simulink model "Standalone_AutoTuner"  (R2025b)
settings: Solver=FixedStepDiscrete  StartTime=0.0  StopTime=20  FixedStep=1e-4  MaxStep=1e-4  RelTol=1e-3  EnableMultiTasking=on
settings Model: SimulationMode=software-in-the-loop (sil)  CodeVerificationMode=processor-in-the-loop (pil)  Creator=Harish  LastModifiedBy=Harish
settings OptimizationCC: DefaultParameterBehavior=Inlined  EnhancedBackFolding=on  PassReuseOutputArgsAs=Individual arguments  ZeroExternalMemoryAtStartup=off  ZeroInternalMemoryAtStartup=off  MaxStackSize=64  OptimizeBlockOrder=speed  DifferentSizesBufferReuse=on  OptimizationCustomize=off  EfficientTunableParamExpr=on
settings DebuggingCC: ParameterTunabilityLossMsg=error
settings HardwareCC: ProdBitPerPointer=32.0  ProdBitPerSizeT=32.0  ProdBitPerPtrDiffT=32.0  ProdLargestAtomicInteger=Long  ProdLargestAtomicFloat=Double  ProdWordSize=32.0  ProdLongLongMode=on  ProdHWDeviceType=ARM Compatible->ARM Cortex-M  TargetLargestAtomicInteger=Long  TargetLargestAtomicFloat=Double  TargetIntDivRoundTo=Zero  TargetEndianess=LittleEndian  TargetHWDeviceType=ARM Compatible->ARM Cortex-M
settings SFSimCC: MATLABDynamicMemAlloc=off
settings RTWCC: SystemTargetFile=ert.tlc  TemplateMakefile=ert_default_tmf  GenerateReport=on  Toolchain=MinGW64 | gmake (64-bit Windows)  GenerateCodeMetricsReport=on  Description=Embedded Coder
settings CodeAppCC: ForceParamTrailComments=on  IgnoreCustomStorageClasses=off  OperatorAnnotations=on  SimulinkDataObjDesc=on  SFDataObjDesc=on  InsertBlockDesc=on
settings ERTTargetCC: ExtModeTransport=3.0  ExtModeStaticAlloc=on  ExtModeStaticAllocSize=2048.0  ExtModeMexFile=ext_xcp  ExtModeIntrfLevel=Level2 - Open  ERTCustomFileTemplate=example_file_process.tlc  TargetLangStandard=C99 (ISO)  CodeReplacementLibrary=ARM Cortex-M  SupportContinuousTime=on

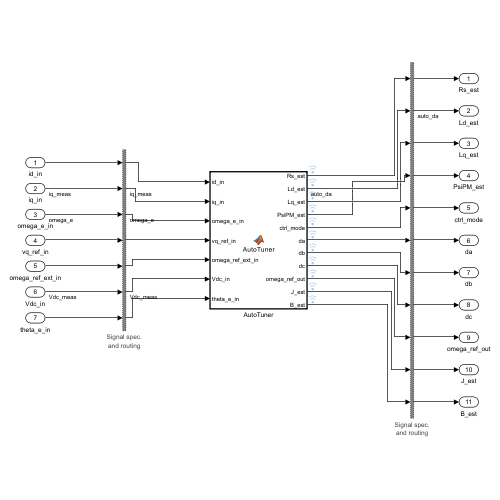
[thumbnail: Simulink's stored preview of the top-level diagram]
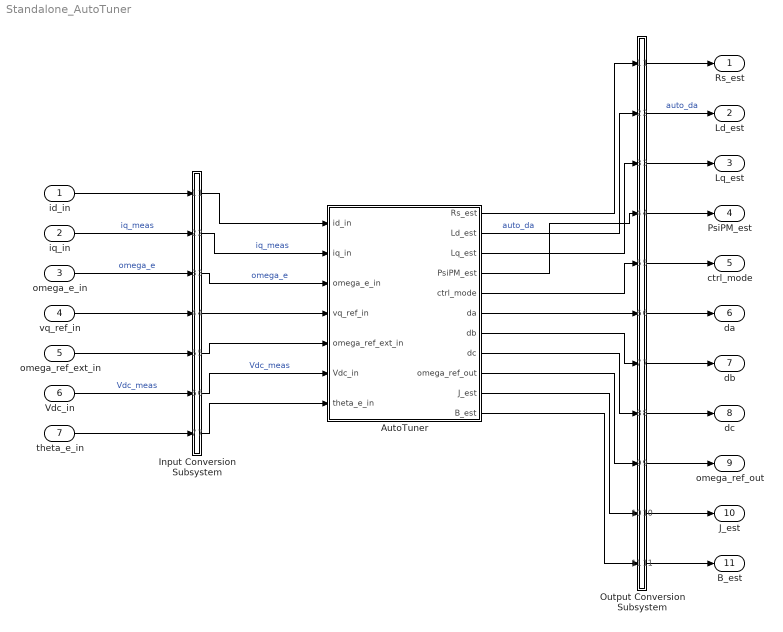
== system Standalone_AutoTuner ==
  id_in : Inport  OutDataTypeStr=double  PortDimensions=[1]  SampleTime=1e-4
  iq_in : Inport  Port=2  OutDataTypeStr=double  PortDimensions=[1]  SampleTime=1e-4
  omega_e_in : Inport  Port=3  OutDataTypeStr=double  PortDimensions=[1]  SampleTime=1e-4
  vq_ref_in : Inport  Port=4  OutDataTypeStr=double  PortDimensions=[1]  SampleTime=1e-4
  omega_ref_ext_in : Inport  Port=5  OutDataTypeStr=double  PortDimensions=[1]  SampleTime=1e-4
  Vdc_in : Inport  Port=6  OutDataTypeStr=double  PortDimensions=[1]  SampleTime=1e-4
  theta_e_in : Inport  Port=7  OutDataTypeStr=double  PortDimensions=[1]  SampleTime=1e-4
  AutoTuner : MATLAB Function  TreatAsAtomicUnit=on
  Input Conversion Subsystem : Subsystem  Tag=__SLT_ICS__  Description=|
      | Signal spec.
      | and routing
      settings: AttributesFormatString=%<Description>
  Output Conversion Subsystem : Subsystem  Tag=__SLT_OCS__  Description=|
      | Signal spec.
      | and routing
      settings: AttributesFormatString=%<Description>
  Rs_est : Outport
  Ld_est : Outport  Port=2
  Lq_est : Outport  Port=3
  PsiPM_est : Outport  Port=4
  ctrl_mode : Outport  Port=5
  da : Outport  Port=6
  db : Outport  Port=7
  dc : Outport  Port=8
  omega_ref_out : Outport  Port=9
  J_est : Outport  Port=10
  B_est : Outport  Port=11
  wires:
  id_in/1 -> Input Conversion Subsystem/1(Inport_1)
  iq_in/1 -> Input Conversion Subsystem/2(Inport_2)  "iq_meas"
  omega_e_in/1 -> Input Conversion Subsystem/3(Inport_3)  "omega_e"
  vq_ref_in/1 -> Input Conversion Subsystem/4(Inport_4)
  omega_ref_ext_in/1 -> Input Conversion Subsystem/5(Inport_5)
  Vdc_in/1 -> Input Conversion Subsystem/6(Inport_6)  "Vdc_meas"
  theta_e_in/1 -> Input Conversion Subsystem/7(Inport_7)
  Output Conversion Subsystem/1(Outport_1) -> Rs_est/1
  Output Conversion Subsystem/2(Outport_2) -> Ld_est/1  "auto_da"
  Output Conversion Subsystem/3(Outport_3) -> Lq_est/1
  Output Conversion Subsystem/4(Outport_4) -> PsiPM_est/1
  Output Conversion Subsystem/5(Outport_5) -> ctrl_mode/1
  Output Conversion Subsystem/6(Outport_6) -> da/1
  Output Conversion Subsystem/7(Outport_7) -> db/1
  Output Conversion Subsystem/8(Outport_8) -> dc/1
  Output Conversion Subsystem/9(Outport_9) -> omega_ref_out/1
  Output Conversion Subsystem/10(Outport_10) -> J_est/1
  Output Conversion Subsystem/11(Outport_11) -> B_est/1
  Input Conversion Subsystem/1(Outport_1) -> AutoTuner/1(id_in)
  Input Conversion Subsystem/2(Outport_2) -> AutoTuner/2(iq_in)  "iq_meas"
  Input Conversion Subsystem/3(Outport_3) -> AutoTuner/3(omega_e_in)  "omega_e"
  Input Conversion Subsystem/4(Outport_4) -> AutoTuner/4(vq_ref_in)
  Input Conversion Subsystem/5(Outport_5) -> AutoTuner/5(omega_ref_ext_in)
  Input Conversion Subsystem/6(Outport_6) -> AutoTuner/6(Vdc_in)  "Vdc_meas"
  Input Conversion Subsystem/7(Outport_7) -> AutoTuner/7(theta_e_in)
  AutoTuner/1(Rs_est) -> Output Conversion Subsystem/1(Inport_1)
  AutoTuner/2(Ld_est) -> Output Conversion Subsystem/2(Inport_2)  "auto_da"
  AutoTuner/3(Lq_est) -> Output Conversion Subsystem/3(Inport_3)
  AutoTuner/4(PsiPM_est) -> Output Conversion Subsystem/4(Inport_4)
  AutoTuner/5(ctrl_mode) -> Output Conversion Subsystem/5(Inport_5)
  AutoTuner/6(da) -> Output Conversion Subsystem/6(Inport_6)
  AutoTuner/7(db) -> Output Conversion Subsystem/7(Inport_7)
  AutoTuner/8(dc) -> Output Conversion Subsystem/8(Inport_8)
  AutoTuner/9(omega_ref_out) -> Output Conversion Subsystem/9(Inport_9)
  AutoTuner/10(J_est) -> Output Conversion Subsystem/10(Inport_10)
  AutoTuner/11(B_est) -> Output Conversion Subsystem/11(Inport_11)

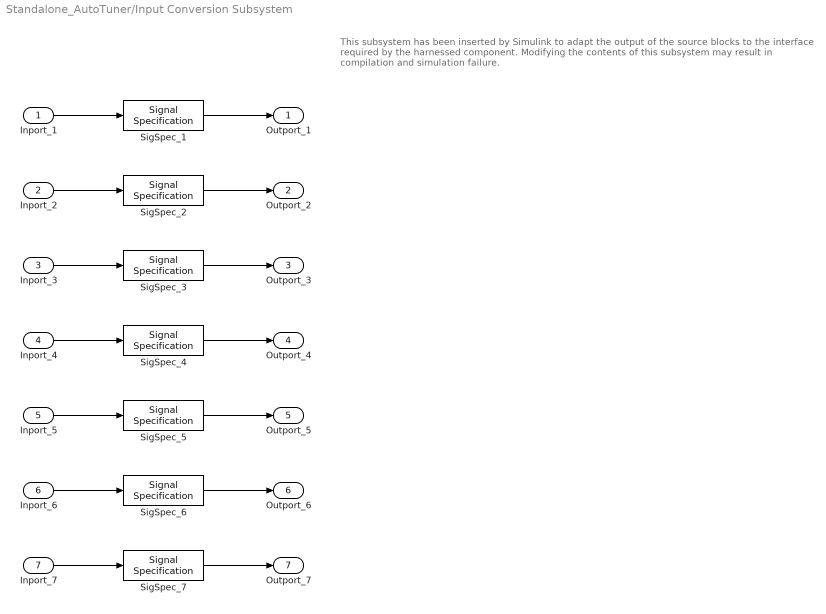
== system Standalone_AutoTuner/Input Conversion Subsystem ==
  note: This subsystem has been inserted by Simulink to adapt the output of the source blocks to the interface required by the harnessed component.
      |  Modifying the contents of this subsystem may result in compilation and simulation failure.
  Inport_1 : Inport
  Inport_2 : Inport  Port=2
  Inport_3 : Inport  Port=3
  Inport_4 : Inport  Port=4
  Inport_5 : Inport  Port=5
  Inport_6 : Inport  Port=6
  Inport_7 : Inport  Port=7
  SigSpec_{1..7} (7 alike) : SignalSpecification  OutDataTypeStr=double  Dimensions=[1]
  Outport_1 : Outport
  Outport_2 : Outport  Port=2
  Outport_3 : Outport  Port=3
  Outport_4 : Outport  Port=4
  Outport_5 : Outport  Port=5
  Outport_6 : Outport  Port=6
  Outport_7 : Outport  Port=7
  wires:
  SigSpec_1/1 -> Outport_1/1
  Inport_1/1 -> SigSpec_1/1
  SigSpec_2/1 -> Outport_2/1
  Inport_2/1 -> SigSpec_2/1
  SigSpec_3/1 -> Outport_3/1
  Inport_3/1 -> SigSpec_3/1
  SigSpec_4/1 -> Outport_4/1
  Inport_4/1 -> SigSpec_4/1
  SigSpec_5/1 -> Outport_5/1
  Inport_5/1 -> SigSpec_5/1
  SigSpec_6/1 -> Outport_6/1
  Inport_6/1 -> SigSpec_6/1
  SigSpec_7/1 -> Outport_7/1
  Inport_7/1 -> SigSpec_7/1

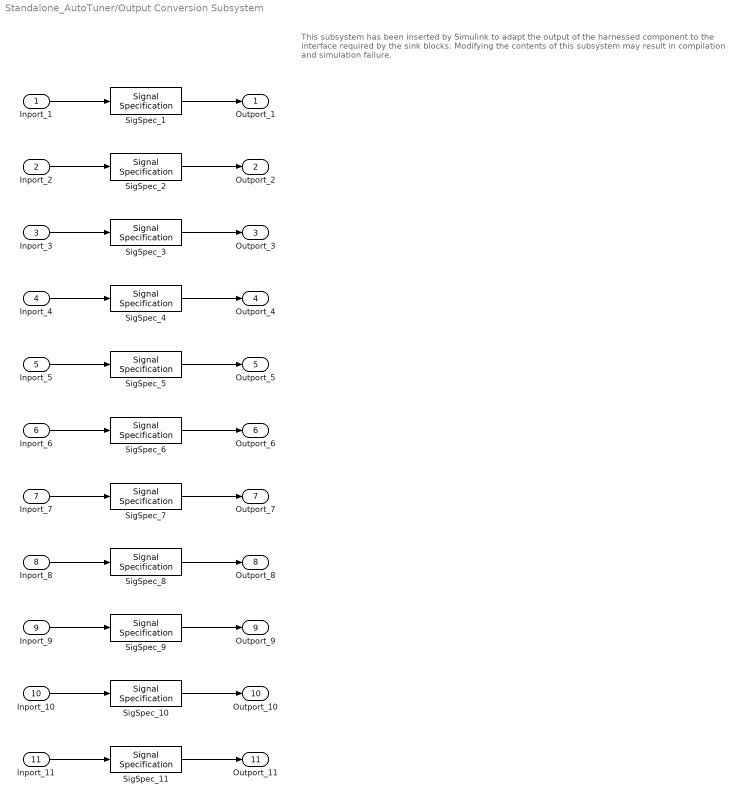
== system Standalone_AutoTuner/Output Conversion Subsystem ==
  note: This subsystem has been inserted by Simulink to adapt the output of the harnessed component to the interface required by the sink blocks.
      |  Modifying the contents of this subsystem may result in compilation and simulation failure.
  Inport_1 : Inport
  Inport_2 : Inport  Port=2
  Inport_3 : Inport  Port=3
  Inport_4 : Inport  Port=4
  Inport_5 : Inport  Port=5
  Inport_6 : Inport  Port=6
  Inport_7 : Inport  Port=7
  Inport_8 : Inport  Port=8
  Inport_9 : Inport  Port=9
  Inport_10 : Inport  Port=10
  Inport_11 : Inport  Port=11
  SigSpec_{1..11} (11 alike) : SignalSpecification  OutDataTypeStr=double  Dimensions=[1]
  Outport_1 : Outport
  Outport_2 : Outport  Port=2
  Outport_3 : Outport  Port=3
  Outport_4 : Outport  Port=4
  Outport_5 : Outport  Port=5
  Outport_6 : Outport  Port=6
  Outport_7 : Outport  Port=7
  Outport_8 : Outport  Port=8
  Outport_9 : Outport  Port=9
  Outport_10 : Outport  Port=10
  Outport_11 : Outport  Port=11
  wires:
  Inport_1/1 -> SigSpec_1/1
  SigSpec_1/1 -> Outport_1/1
  Inport_2/1 -> SigSpec_2/1
  SigSpec_2/1 -> Outport_2/1
  Inport_3/1 -> SigSpec_3/1
  SigSpec_3/1 -> Outport_3/1
  Inport_4/1 -> SigSpec_4/1
  SigSpec_4/1 -> Outport_4/1
  Inport_5/1 -> SigSpec_5/1
  SigSpec_5/1 -> Outport_5/1
  Inport_6/1 -> SigSpec_6/1
  SigSpec_6/1 -> Outport_6/1
  Inport_7/1 -> SigSpec_7/1
  SigSpec_7/1 -> Outport_7/1
  Inport_8/1 -> SigSpec_8/1
  SigSpec_8/1 -> Outport_8/1
  Inport_9/1 -> SigSpec_9/1
  SigSpec_9/1 -> Outport_9/1
  Inport_10/1 -> SigSpec_10/1
  SigSpec_10/1 -> Outport_10/1
  Inport_11/1 -> SigSpec_11/1
  SigSpec_11/1 -> Outport_11/1

== matlab function Standalone_AutoTuner/AutoTuner ==
  settings: updateMethod=DISCRETE  sampleTime=Ts_ctrl
  data: Rs_est output size=1; Ld_est output size=1; Lq_est output size=1; PsiPM_est output size=1; id_in input; iq_in input; omega_e_in input; vq_ref_in input; omega_ref_ext_in input; Vdc_in input; ctrl_mode output; da output; db output; dc output; omega_ref_out output; J_est output; B_est output; theta_e_in input
function [Rs_est, Ld_est, Lq_est, PsiPM_est, ctrl_mode, da, db, dc, omega_ref_out, J_est, B_est] = ...
    AutoTuner(id_in, iq_in, omega_e_in, vq_ref_in, omega_ref_ext_in, Vdc_in, theta_e_in)
    
    % ====================================================================
    % 1. USER CONFIGURATION BLOCK
    % ====================================================================
    I_MAX_RATING = 565.0;  % Peak phase current of the motor (Amps)
    V_DC_NOMINAL = 400.0;  % Nominal DC link voltage (Volts)
    W_MIN_FLUX   = 800.0;  % Speed required for clean Back-EMF reading
    POLE_PAIRS   = 6.0;    % REQUIRED FOR MECHANICAL MATH: Number of pole pairs
    
    I_SPIN_FLUX = 0.10 * I_MAX_RATING; 
    V_HF_AMP    = 0.04 * V_DC_NOMINAL; 
    % ====================================================================
    persistent state sub_state count state_timer
    persistent int_err_d int_err_q
    persistent Rs_val Ld_val Lq_val PsiPM_val J_val B_val
    persistent V_sum I_sum sample_k 
    persistent Vd1 Id1 I_sin I_cos
    persistent Kp_calc Ki_calc 
    persistent Vd_bias 
    
    % Mechanical estimation persistent variables
    persistent w_start w_start_sum int_err_spd Te_1 w_1
    
    % --- Explicitly initialize outputs for Simulink Coder ---
    Rs_est = 0.0; Ld_est = 0.0; Lq_est = 0.0; PsiPM_est = 0.0;
    ctrl_mode = 0.0; da = 0.0; db = 0.0; dc = 0.0;
    omega_ref_out = 0.0; J_est = 0.0; B_est = 0.0;
    
    Ts = 1e-4;   % Sample time (10 kHz)
    f_hf = 500;  
    w_hf = 2 * pi * f_hf;
    
    if isempty(state)
        state = 0; sub_state = 0; count = 0; state_timer = 0; 
        int_err_d = 0; int_err_q = 0;
        Rs_val = 0.005; Ld_val = 0.0001; Lq_val = 0.0001; PsiPM_val = 0.04;
        J_val = 0.0; B_val = 0.0; 
        V_sum = 0; I_sum = 0; sample_k = 0; 
        Vd1 = 0; Id1 = 0; I_sin = 0; I_cos = 0;
        Kp_calc = 0.1; Ki_calc = 10; 
        Vd_bias = 0;
        w_start = 0; w_start_sum = 0; int_err_spd = 0; Te_1 = 0; w_1 = 0;
    end
    
    t = double(count) * Ts;
    id = double(id_in); iq = double(iq_in); omega_e = double(omega_e_in); 
    Vdc = double(Vdc_in); theta_e = double(theta_e_in);
    omega_ref_ext = double(omega_ref_ext_in);
    
    Vd_applied = 0; Vq_applied = 0;
    
    V_limit = Vdc / 1.5; 
    if V_limit < 1, V_limit = 24; end 
    %% --- DYNAMIC STATE MACHINE ---
    
    if state == 0 % --- STATE 0: Pulse Test for Dynamic PI Tuning ---
        ctrl_mode = 2; 
        
        V_pulse = V_HF_AMP; 
        Vd_applied = V_pulse;
        Vq_applied = 0;
        
        if sample_k == 0
            Id1 = id; 
        end
        
        sample_k = sample_k + 1;
        
        if sample_k >= 5 
            di = id - Id1;
            dt = 5 * Ts;
            
            if di < 0.1, di = 0.1; end 
            
            L_rough = (V_pulse * dt) / di;
            omega_bw = 1000; 
            
            Kp_calc = L_rough * omega_bw;
            Ki_calc = Kp_calc * 100; 
            
            if Kp_calc > 2.0, Kp_calc = 2.0; end
            if Kp_calc < 0.001, Kp_calc = 0.001; end
            
            state = 1; sub_state = 0; state_timer = t;
            sample_k = 0; V_sum = 0; I_sum = 0; Id1 = 0;
        end
        
    elseif state == 1 % --- Identify Stator Resistance (Rs) ---
        ctrl_mode = 2; 
        iq_ref = 0;
        
        if sub_state == 0
            id_ref = 0.10 * I_MAX_RATING; 
            
            err_d = id_ref - id; err_q = iq_ref - iq;
            int_err_d = max(min(int_err_d + err_d * Ts, V_limit/Ki_calc), -V_limit/Ki_calc);
            int_err_q = max(min(int_err_q + err_q * Ts, V_limit/Ki_calc), -V_limit/Ki_calc);
            
            Vd_applied = Kp_calc * err_d + Ki_calc * int_err_d;
            Vq_applied = Kp_calc * err_q + Ki_calc * int_err_q;
            
            if (t - state_timer) > 0.4
                V_sum = V_sum + Vd_applied;
                I_sum = I_sum + id;
                sample_k = sample_k + 1;
            end
            
            if sample_k >= 100
                Vd1 = V_sum / sample_k;
                Id1 = I_sum / sample_k;
                sub_state = 1; state_timer = t;
                V_sum = 0; I_sum = 0; sample_k = 0;
            end
            
        elseif sub_state == 1
            id_ref = 0.20 * I_MAX_RATING; 
            
            err_d = id_ref - id; err_q = iq_ref - iq;
            int_err_d = max(min(int_err_d + err_d * Ts, V_limit/Ki_calc), -V_limit/Ki_calc);
            int_err_q = max(min(int_err_q + err_q * Ts, V_limit/Ki_calc), -V_limit/Ki_calc);
            
            Vd_applied = Kp_calc * err_d + Ki_calc * int_err_d;
            Vq_applied = Kp_calc * err_q + Ki_calc * int_err_q;
            
            if (t - state_timer) > 0.4
                V_sum = V_sum + Vd_applied;
                I_sum = I_sum + id;
                sample_k = sample_k + 1;
            end
            
            if sample_k >= 100
                Vd2 = V_sum / sample_k;
                Id2 = I_sum / sample_k;
                if abs(Id2 - Id1) > 1.0
                    Rs_val = (Vd2 - Vd1) / (Id2 - Id1); if Rs_val < 0.0001, Rs_val = 0.0001; end 
                end
                state = 2; state_timer = t; sub_state = 0;
                int_err_d = 0; int_err_q = 0;
                V_sum = 0; I_sum = 0; sample_k = 0;
            end
        end
        
    elseif state == 2 % --- Identify d-axis Inductance (Ld) ---
        ctrl_mode = 2; 
        
        iq_ref = 0;
        err_q = iq_ref - iq;
        int_err_q = max(min(int_err_q + err_q * Ts, V_limit/Ki_calc), -V_limit/Ki_calc);
        Vq_applied = Kp_calc * err_q + Ki_calc * int_err_q; 
        
        if sub_state == 0
            id_ref = 0.10 * I_MAX_RATING;
            err_d = id_ref - id;
            int_err_d = max(min(int_err_d + err_d * Ts, V_limit/Ki_calc), -V_limit/Ki_calc);
            Vd_applied = Kp_calc * err_d + Ki_calc * int_err_d;
            
            if (t - state_timer) > 0.4
                Vd_bias = Vd_applied; 
                sub_state = 1;
                state_timer = t;
                sample_k = 0; I_sin = 0; I_cos = 0;
            end
            
        elseif sub_state == 1
            Vd_applied = Vd_bias + V_HF_AMP * sin(w_hf * t);
            
            if (t - state_timer) > 0.2
                I_sin = I_sin + id * sin(w_hf * t);
                I_cos = I_cos + id * cos(w_hf * t);
                sample_k = sample_k + 1;
            end
            
            if sample_k >= 200
                I_hf_amp = (2 * sqrt(I_sin^2 + I_cos^2)) / sample_k;
                
                if I_hf_amp > 0.01 
                    Z = V_HF_AMP / I_hf_amp;
                    if Z > Rs_val, Ld_val = sqrt(max(0, Z^2 - Rs_val^2)) / w_hf;
                    else,          Ld_val = Z / w_hf; end
                end
                state = 3; state_timer = t; sub_state = 0;
                int_err_d = 0; int_err_q = 0; 
                I_sin = 0; I_cos = 0; sample_k = 0;
            end
        end
        
    elseif state == 3 % --- Identify q-axis Inductance (Lq) ---
        ctrl_mode = 2; 
        id_ref = 0;
        
        err_d = id_ref - id;
        int_err_d = max(min(int_err_d + err_d * Ts, V_limit/Ki_calc), -V_limit/Ki_calc);
        
        Vd_applied = Kp_calc * err_d + Ki_calc * int_err_d;
        Vq_applied = V_HF_AMP * sin(w_hf * t);
        
        if (t - state_timer) > 0.2
            I_sin = I_sin + iq * sin(w_hf * t);
            I_cos = I_cos + iq * cos(w_hf * t);
            sample_k = sample_k + 1;
        end
        
        if sample_k >= 200
            I_hf_amp = (2 * sqrt(I_sin^2 + I_cos^2)) / sample_k;
            
            if I_hf_amp > 0.01
                Z = V_HF_AMP / I_hf_amp;
                if Z > Rs_val, Lq_val = sqrt(max(0, Z^2 - Rs_val^2)) / w_hf;
                else,          Lq_val = Z / w_hf; end
            end
            state = 4; state_timer = t; sub_state = 0;
            int_err_d = 0; int_err_q = 0; 
            I_sin = 0; I_cos = 0; sample_k = 0; V_sum = 0;
        end
        
    elseif state == 4 % --- Identify PM Flux Linkage (PsiPM) ---
        ctrl_mode = 2; 
        
        if sub_state == 0
            id_ref = 0; 
            iq_ref = I_SPIN_FLUX; 
            
            err_d = id_ref - id; err_q = iq_ref - iq;
            int_err_d = max(min(int_err_d + err_d * Ts, V_limit/Ki_calc), -V_limit/Ki_calc);
            int_err_q = max(min(int_err_q + err_q * Ts, V_limit/Ki_calc), -V_limit/Ki_calc);
            
            Vd_applied = Kp_calc * err_d + Ki_calc * int_err_d;
            Vq_applied = Kp_calc * err_q + Ki_calc * int_err_q;
            
            if abs(omega_e) > W_MIN_FLUX
                sub_state = 1; 
                state_timer = t; 
            end
            
        elseif sub_state == 1
            id_ref = 0; 
            iq_ref = 0; 
            
            err_d = id_ref - id; err_q = iq_ref - iq;
            int_err_d = max(min(int_err_d + err_d * Ts, V_limit/Ki_calc), -V_limit/Ki_calc);
            int_err_q = max(min(int_err_q + err_q * Ts, V_limit/Ki_calc), -V_limit/Ki_calc);
            
            Vd_applied = Kp_calc * err_d + Ki_calc * int_err_d;
            Vq_applied = Kp_calc * err_q + Ki_calc * int_err_q;
            
            if (t - state_timer) > 0.5
                if abs(omega_e) > (W_MIN_FLUX / 2) 
                    inst_psi = Vq_applied / omega_e;
                    V_sum = V_sum + inst_psi;
                    sample_k = sample_k + 1;
                end
            end
            
            if sample_k >= 200
                PsiPM_val = V_sum / sample_k;
                state = 5; sub_state = 0; state_timer = t; 
                sample_k = 0; I_sum = 0; w_start_sum = 0; 
                int_err_spd = 0;
            end
        end
        
    elseif state == 5 % --- Identify Friction (B) and Inertia (J) [Two-Point Method] ---
        ctrl_mode = 2; 
        
        if sub_state == 0 % Point 1: Settle at 60 rad/s
            w_mech = omega_e / POLE_PAIRS;
            w_target = 60.0; 
            
            % Automatically scale PI gains based on the motor's power class
            Kp_spd = 0.005 * I_MAX_RATING; 
            Ki_spd = 0.020 * I_MAX_RATING; 
            
            err_spd = w_target - w_mech;
            int_err_spd = max(min(int_err_spd + err_spd * Ts, I_SPIN_FLUX/Ki_spd), -I_SPIN_FLUX/Ki_spd);
            
            iq_ref = Kp_spd * err_spd + Ki_spd * int_err_spd;
            iq_ref = max(min(iq_ref, I_SPIN_FLUX), -I_SPIN_FLUX); 
            id_ref = 0; 
            
            err_d = id_ref - id; err_q = iq_ref - iq;
            int_err_d = max(min(int_err_d + err_d * Ts, V_limit/Ki_calc), -V_limit/Ki_calc);
            int_err_q = max(min(int_err_q + err_q * Ts, V_limit/Ki_calc), -V_limit/Ki_calc);
            
            Vd_applied = Kp_calc * err_d + Ki_calc * int_err_d;
            Vq_applied = Kp_calc * err_q + Ki_calc * int_err_q;
            
            % STRICT ABSOLUTE TIMER: Wait 1.5s to guarantee acceleration is identically zero.
            if (t - state_timer) > 1.5
                sample_k = sample_k + 1;
                
                % Use the mathematically clean commanded current (iq_ref), not noisy feedback
                I_sum = I_sum + iq_ref; 
                w_start_sum = w_start_sum + w_mech;
                
                if sample_k >= 250 
                    iq_avg = I_sum / 250.0;
                    w_1 = w_start_sum / 250.0;
                    Te_1 = 1.5 * POLE_PAIRS * PsiPM_val * iq_avg;
                    
                    sub_state = 1; state_timer = t; 
                    sample_k = 0; I_sum = 0; w_start_sum = 0; 
                    int_err_spd = 0; int_err_q = 0;
                end
            end
            
        elseif sub_state == 1 % Point 2: Settle at 120 rad/s
            w_mech = omega_e / POLE_PAIRS;
            w_target = 120.0; 
            
            Kp_spd = 0.005 * I_MAX_RATING; 
            Ki_spd = 0.020 * I_MAX_RATING; 
            
            err_spd = w_target - w_mech;
            int_err_spd = max(min(int_err_spd + err_spd * Ts, I_SPIN_FLUX/Ki_spd), -I_SPIN_FLUX/Ki_spd);
            
            iq_ref = Kp_spd * err_spd + Ki_spd * int_err_spd;
            iq_ref = max(min(iq_ref, I_SPIN_FLUX), -I_SPIN_FLUX); 
            id_ref = 0; 
            
            err_d = id_ref - id; err_q = iq_ref - iq;
            int_err_d = max(min(int_err_d + err_d * Ts, V_limit/Ki_calc), -V_limit/Ki_calc);
            int_err_q = max(min(int_err_q + err_q * Ts, V_limit/Ki_calc), -V_limit/Ki_calc);
            
            Vd_applied = Kp_calc * err_d + Ki_calc * int_err_d;
            Vq_applied = Kp_calc * err_q + Ki_calc * int_err_q;
            
            % STRICT ABSOLUTE TIMER: Wait 1.5s to guarantee acceleration is identically zero.
            if (t - state_timer) > 1.5
                sample_k = sample_k + 1;
                
                % Use the mathematically clean commanded current (iq_ref)
                I_sum = I_sum + iq_ref; 
                w_start_sum = w_start_sum + w_mech;
                
                if sample_k >= 250 
                    iq_avg = I_sum / 250.0;
                    w_2 = w_start_sum / 250.0;
                    Te_2 = 1.5 * POLE_PAIRS * PsiPM_val * iq_avg;
                    
                    if abs(w_2 - w_1) > 10.0
                        B_val = abs(Te_2 - Te_1) / abs(w_2 - w_1); 
                    end
                    
                    if B_val <= 0, B_val = 0.0001; end 
                    
                    sub_state = 2; state_timer = t; 
                    sample_k = 0; int_err_q = 0; int_err_spd = 0;
                end
            end
            
        elseif sub_state == 2 % Point 3: Active Braking Step (Identify Inertia J)
            id_ref = 0; 
            iq_ref = -I_SPIN_FLUX; 
            
            err_d = id_ref - id; err_q = iq_ref - iq;
            int_err_d = max(min(int_err_d + err_d * Ts, V_limit/Ki_calc), -V_limit/Ki_calc);
            int_err_q = max(min(int_err_q + err_q * Ts, V_limit/Ki_calc), -V_limit/Ki_calc);
            
            Vd_applied = Kp_calc * err_d + Ki_calc * int_err_d;
            Vq_applied = Kp_calc * err_q + Ki_calc * int_err_q;
            
            if (t - state_timer) > 0.1
                if sample_k == 0
                    w_start = omega_e / POLE_PAIRS;
                end
                
                sample_k = sample_k + 1;
                
                if sample_k >= 100
                    w_end = omega_e / POLE_PAIRS;
                    dw_dt = (w_end - w_start) / (100 * Ts);
                    w_avg = (w_end + w_start) / 2;
                    
                    % Use the clean commanded current for the torque calculation
                    Te = 1.5 * POLE_PAIRS * PsiPM_val * iq_ref;
                    
                    if abs(dw_dt) > 1e-4
                        J_val = abs(Te - (B_val * w_avg)) / abs(dw_dt); 
                    else
                        J_val = 0.0867; 
                    end
                    
                    if J_val <= 0.0001, J_val = 0.001; end 
                    
                    state = 6; 
                end
            end
        end
        
    elseif state == 6 % --- Mission Profile ---
        ctrl_mode = 1; 
        da = 0.5; db = 0.5; dc = 0.5; 
        omega_ref_out = omega_ref_ext;
    end
    
    %% --- INVERSE PARK & SPACE VECTOR MODULATION ---
    if state < 6
        valpha = Vd_applied * cos(theta_e) - Vq_applied * sin(theta_e);
        vbeta  = Vd_applied * sin(theta_e) + Vq_applied * cos(theta_e);
        
        va = valpha; 
        vb = -0.5 * valpha + 0.8660254 * vbeta; 
        vc = -0.5 * valpha - 0.8660254 * vbeta;
        
        voff = -0.5 * (max([va, vb, vc]) + min([va, vb, vc]));
        
        da = (va + voff) / (Vdc / 2) * 0.5 + 0.5;
        db = (vb + voff) / (Vdc / 2) * 0.5 + 0.5;
        dc = (vc + voff) / (Vdc / 2) * 0.5 + 0.5;
        
        da = max(min(da, 1), 0);
        db = max(min(db, 1), 0);
        dc = max(min(dc, 1), 0);
    end
    
    %% --- OUTPUT ASSIGNMENT ---
    Rs_est = Rs_val; 
    Ld_est = Ld_val; 
    Lq_est = Lq_val; 
    PsiPM_est = PsiPM_val;
    J_est = J_val; 
    B_est = B_val;
    
    count = count + 1;
end
